simulink model "e2c"  (R2021a)
settings: Solver=VariableStepAuto  StartTime=0.0  StopTime=10.0  RelTol=1e-3
undefined symbols (not defined in the file): Rec, SDTV
libraries: visionconversions x2, visionsources x1
settings Model: Creator=pranshu  LastModifiedBy=pranshu

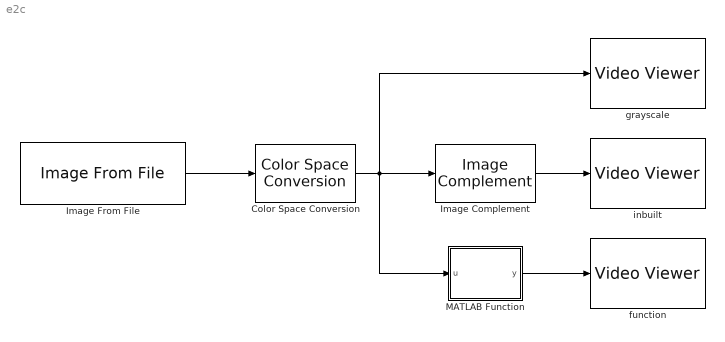
== system e2c ==
  Color Space Conversion : visionconversions/Color Space  Conversion  conversion=Obsolete  conversionActive=R'G'B' to intensity  wp_str=D65  rec=Rec. 601 (SDTV)  sys=1125/60/2:1  imagePorts=One multidimensional signal
  Image Complement : visionconversions/Image Complement
      settings: SourceProductBaseCode=VP
  Image From File : visionsources/Image From File  Tag=vipblks_nd  FileName=peppers.png  Ts=inf  imagePorts=One multidimensional signal  OutPortLabels=R|G|B  ImageDataType=Inherit from input image  sdImageDataType=uint(8)  Signed=on  WordLength=16  FractionLengthMode=User-defined  FractionLength=15
  MATLAB Function : MATLAB Function  TreatAsAtomicUnit=on
  function : VideoViewer  FigPos=[2041 741 418 304]
  grayscale : VideoViewer  FigPos=[2041 741 418 304]
  inbuilt : VideoViewer  FigPos=[2041 741 418 304]
  wires:
  MATLAB Function/1(y) -> function/1
  Color Space Conversion/1 -> Image Complement/1, MATLAB Function/1(u), grayscale/1
  Image Complement/1 -> inbuilt/1
  Image From File/1 -> Color Space Conversion/1

== matlab function e2c/MATLAB Function ==
  data: u input; y output
function y = fcn(u)
y=u;
for r=1:size(u,1)
    for c=1:size(u,2)
        y(r,c)=255-u(r,c);
    end
end
